simulink library "quat_degerr_lib"  (R2018b)
settings: Solver=VariableStepAuto  StartTime=0.0  StopTime=10.0  RelTol=1e-3
undefined symbols (not defined in the file or in its folder): fswParams
libraries: aerolibutil x2
settings Model: Creator=Taylor  LastModifiedBy=taylorreynolds

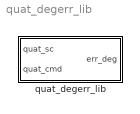
== system quat_degerr_lib ==
  quat_degerr_lib : Subsystem

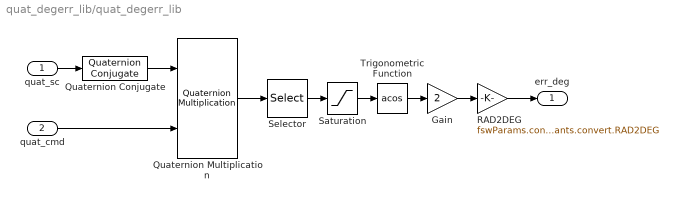
== system quat_degerr_lib/quat_degerr_lib ==
  quat_sc : Inport
  quat_cmd : Inport  Port=2
  Gain : Gain  Gain=2
  Quaternion Conjugate : aerolibutil/Quaternion Conjugate
      settings: SourceProductName=Aerospace Blockset  SourceProductBaseCode=AE
  Quaternion Multiplication : aerolibutil/Quaternion Multiplication
  RAD2DEG : Gain  Gain=fswParams.constants.convert.RAD2DEG
  Saturation : Saturate  UpperLimit=1  LowerLimit=-1
  Selector : Selector  InputPortWidth=4  IndexOptions=Index vector (dialog)  Indices=1  OutputSizes=1
  Trigonometric Function : Trigonometry  Operator=acos
  err_deg : Outport
  wires:
  quat_cmd/1 -> Quaternion Multiplication/2
  Saturation/1 -> Trigonometric Function/1
  Quaternion Multiplication/1 -> Selector/1
  Trigonometric Function/1 -> Gain/1
  Gain/1 -> RAD2DEG/1
  Selector/1 -> Saturation/1
  Quaternion Conjugate/1 -> Quaternion Multiplication/1
  quat_sc/1 -> Quaternion Conjugate/1
  RAD2DEG/1 -> err_deg/1
